simulink model "RBG_einMassenmodell_Versuchsplanung"  (Simulink 9.0)
settings: Solver=ode45  StartTime=0.0  StopTime=30  MaxStep=0.02  RelTol=1e-3  EnableMultiTasking=on
values from neighbouring files (symbols this model uses):
  hubMatlab = hubTest(k)    [generateErgebniseTabelle.m]    (also in simData.mat = 22)
  lastMatlab = masseTest(j)    [generateErgebniseTabelle.m]    (also in simData.mat = 560)
  zeitMatlab = zeitTest(l)    [generateErgebniseTabelle.m]    (also in simData.mat = 30)
libraries: simulink x1
settings Model: SuppressorTable=22 serialization::archive 11 0 6 0 0 0 11 0  Creator=beck  LastModifiedBy=jens
settings DataIOCC: LimitDataPoints=on  SignalLoggingSaveFormat=ModelDataLogs
settings OptimizationCC: ExpressionDepthLimit=2147483647  InitFltsAndDblsToZero=on
settings DebuggingCC: SaveWithParameterizedLinksMsg=none  SignalResolutionControl=TryResolveAllWithWarning  SolverPrmCheckMsg=warning  FcnCallInpInsideContextMsg=warning  StateNameClashWarn=warning  StrictBusMsg=Warning
settings GRTTargetCC: TargetFcnLib=ansi_tfl_tmw.mat  GeneratePreprocessorConditionals=Disable all  CombineOutputUpdateFcns=off  GRTInterface=on

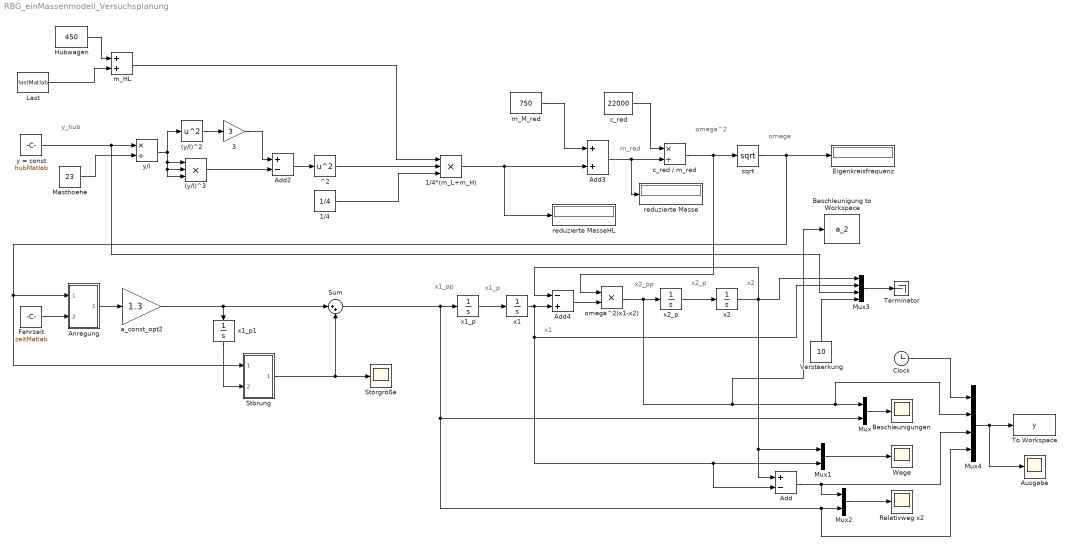
== system RBG_einMassenmodell_Versuchsplanung ==
  note: y_hub
  note: m_red
  note: omega^2
  note: x1_pp
  note: x2_pp
  note: x2_p
  note: x1_p
  note: omega
  note: x2
  note: x1
  (y/l)^2 : Math  Operator=square  SaturateOnIntegerOverflow=on
  (y/l)^3 : Product  Inputs=3  RndMeth=Zero
  1/4 : Constant  Value=1/4
  1/4*(m_L+m_H) : Product  Inputs=3  RndMeth=Zero
  3 : Gain  Gain=3
  Add : Sum  Inputs=+-
  Add2 : Sum  Inputs=+-
  Add3 : Sum
  Add4 : Sum  Inputs=-+
  Anregung : Subsystem
  Ausgabe : Scope
  Beschleunigung to Workspace : ToWorkspace  VariableName=a_2  SampleTime=-1
      settings: Save2DSignal=2-D array (concatenate along first dimension)
  Beschleunigungen : Scope
  Clock : Clock
  Eigenkreisfrequenz : Display
  Fahrzeit : Constant  Value=zeitMatlab
  Hubwagen : Constant  Value=450
  Last : Constant  Value=lastMatlab
  Masthoehe : Constant  Value=23
  Mux : Mux  Inputs=2
  Mux1 : Mux  Inputs=2
  Mux2 : Mux  Inputs=2
  Mux3 : Mux
  Mux4 : Mux
  Relativweg x2 : Scope
  Störgröße : Scope
  Störung : Subsystem
  Sum : Sum  Inputs=|++
  Terminator : Terminator
  To Workspace : ToWorkspace  VariableName=y  SampleTime=-1
  Verstaerkung : Constant  Value=10
  Wege : Scope
  ^2 : Math  Operator=square  SaturateOnIntegerOverflow=on
  a_const_opt2 : Gain  Gain=1.3
  c_red : Constant  Value=22000
  c_red / m_red : Product  Inputs=*/  RndMeth=Zero
  m_HL : Sum
  m_M_red : Constant  Value=750
  omega^2(x1-x2) : Product  RndMeth=Zero
  reduzierte Masse : Display
  reduzierte MasseHL : Display
  sqrt : Math  Operator=sqrt  SaturateOnIntegerOverflow=on
  x1 : Integrator
  x1_p : Integrator
  x1_p1 : Integrator
  x2 : Integrator
  x2_p : Integrator
  y = const : Constant  Value=hubMatlab
  y/l : Product  Inputs=*/  RndMeth=Zero
  wires:
  y = const/1 -> y/l/1, Mux3/3
  Mux/1 -> Beschleunigungen/1
  Mux1/1 -> Wege/1
  Masthoehe/1 -> y/l/2
  (y/l)^2/1 -> 3/1
  3/1 -> Add2/1
  (y/l)^3/1 -> Add2/2
  y/l/1 -> (y/l)^3/1, (y/l)^3/2, (y/l)^3/3, (y/l)^2/1
  c_red/1 -> c_red / m_red/1
  c_red / m_red/1 -> sqrt/1, omega^2(x1-x2)/1
  Add3/1 -> reduzierte Masse/1, c_red / m_red/2
  sqrt/1 -> Eigenkreisfrequenz/1, Störung/1(In1), Anregung/1(In1)
  omega^2(x1-x2)/1 -> x2_p/1, Beschleunigung to Workspace/1, Mux/1, Mux4/2
  x2_p/1 -> x2/1
  x1_p/1 -> x1/1
  Add4/1 -> omega^2(x1-x2)/2
  x1/1 -> Add4/2, Mux1/2, Add/2, Mux3/2
  x2/1 -> Mux1/1, Add/1, Mux3/1, Add4/1
  Verstaerkung/1 -> Mux3/4
  Add2/1 -> ^2/1
  m_M_red/1 -> Add3/1
  Mux2/1 -> Relativweg x2/1
  Add/1 -> Mux4/3, Mux2/1
  Last/1 -> m_HL/2
  Hubwagen/1 -> m_HL/1
  1/4*(m_L+m_H)/1 -> Add3/2, reduzierte MasseHL/1
  ^2/1 -> 1/4*(m_L+m_H)/2
  m_HL/1 -> 1/4*(m_L+m_H)/1
  1/4/1 -> 1/4*(m_L+m_H)/3
  Sum/1 -> x1_p/1, Mux/2, Mux2/2, Mux4/4
  Anregung/1(Out1) -> a_const_opt2/1
  Störung/1(Out1) -> Störgröße/1, Sum/2
  Clock/1 -> Mux4/1
  Mux4/1 -> To Workspace/1, Ausgabe/1
  a_const_opt2/1 -> Sum/1, x1_p1/1
  x1_p1/1 -> Störung/2(In2)
  Mux3/1 -> Terminator/1
  Fahrzeit/1 -> Anregung/2(In2)

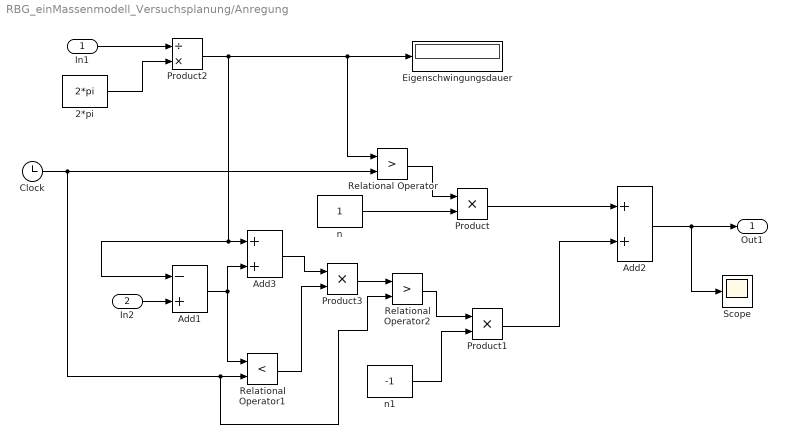
== system RBG_einMassenmodell_Versuchsplanung/Anregung ==
  In1 : Inport
  In2 : Inport  Port=2
  2*pi : Constant  Value=2*pi
  Add1 : Sum  Inputs=-+
  Add2 : Sum
  Add3 : Sum
  Clock : Clock
  Eigenschwingungsdauer : Display
  Product : Product  RndMeth=Zero
  Product1 : Product  RndMeth=Zero
  Product2 : Product  Inputs=/*  RndMeth=Zero
  Product3 : Product  RndMeth=Zero
  Relational Operator : RelationalOperator  Operator=>  RndMeth=Nearest
  Relational Operator1 : RelationalOperator  Operator=<  RndMeth=Nearest
  Relational Operator2 : RelationalOperator  Operator=>  RndMeth=Nearest
  Scope : Scope
  n : Constant
  n1 : Constant  Value=-1
  Out1 : Outport
  wires:
  2*pi/1 -> Product2/2
  Clock/1 -> Relational Operator/2, Relational Operator2/2, Relational Operator1/2
  n/1 -> Product/2
  Product2/1 -> Eigenschwingungsdauer/1, Relational Operator/1, Add1/1, Add3/1
  Relational Operator/1 -> Product/1
  In1/1 -> Product2/1
  Add2/1 -> Out1/1, Scope/1
  Product/1 -> Add2/1
  n1/1 -> Product1/2
  Relational Operator2/1 -> Product1/1
  Add3/1 -> Product3/1
  Relational Operator1/1 -> Product3/2
  Product3/1 -> Relational Operator2/1
  Product1/1 -> Add2/2
  In2/1 -> Add1/2
  Add1/1 -> Relational Operator1/1, Add3/2

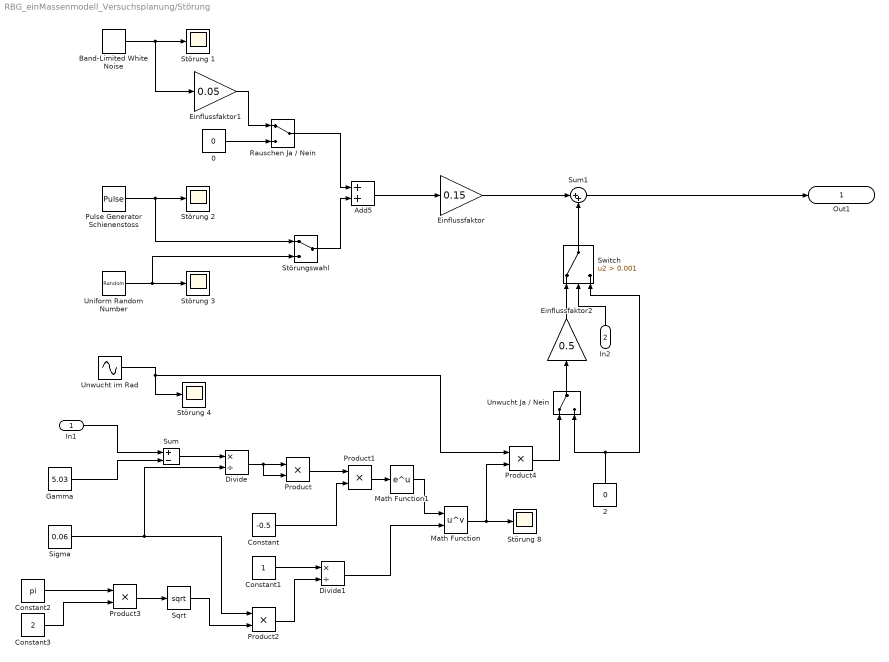
== system RBG_einMassenmodell_Versuchsplanung/Störung ==
  In1 : Inport
  In2 : Inport  Port=2
  0 : Constant  Value=0
  2 : Constant  Value=0
  Add5 : Sum
  Band-Limited White Noise : simulink/Sources/Band-Limited White Noise  Cov=[0.1]  Ts=0.1  seed=[23341]
  Constant : Constant  Value=-0.5
  Constant1 : Constant
  Constant2 : Constant  Value=pi
  Constant3 : Constant  Value=2
  Divide : Product  Inputs=*/
  Divide1 : Product  Inputs=*/
  Einflussfaktor : Gain  Gain=0.15
  Einflussfaktor1 : Gain  Gain=0.05
  Einflussfaktor2 : Gain  Gain=0.5
  Gamma : Constant  Value=5.03
  Math Function : Math  Operator=pow  SaturateOnIntegerOverflow=on
  Math Function1 : Math  SaturateOnIntegerOverflow=on
  Product{,1..4} (5 alike) : Product  RndMeth=Zero
  Pulse Generator Schienenstoss : DiscretePulseGenerator  PulseType=Time based  Amplitude=-1  Period=4
  Rauschen Ja / Nein : ManualSwitch
  Sigma : Constant  Value=0.06
  Sqrt : Sqrt  SaturateOnIntegerOverflow=on
  Störung {1..4,8} (5 alike) : Scope
  Störungswahl : ManualSwitch
  Sum : Sum  Inputs=+-
  Sum1 : Sum  Inputs=|++
  Switch : Switch  Criteria=u2 > Threshold  Threshold=0.001
  Uniform Random Number : UniformRandomNumber  SampleTime=1
  Unwucht Ja / Nein : ManualSwitch
  Unwucht im Rad : Sin  Frequency=5  SampleTime=0
  Out1 : Outport
  wires:
  Pulse Generator Schienenstoss/1 -> Störung 2/1, Störungswahl/1
  Add5/1 -> Einflussfaktor/1
  Band-Limited White Noise/1 -> Störung 1/1, Einflussfaktor1/1
  Störungswahl/1 -> Add5/2
  Uniform Random Number/1 -> Störung 3/1, Störungswahl/2
  Rauschen Ja / Nein/1 -> Add5/1
  Unwucht im Rad/1 -> Störung 4/1, Product4/1
  Gamma/1 -> Sum/2
  Sum/1 -> Divide/1
  Sigma/1 -> Divide/2, Product2/1
  Divide/1 -> Product/1, Product/2
  Product/1 -> Product1/1
  Constant/1 -> Product1/2
  Constant1/1 -> Divide1/1
  Constant2/1 -> Product3/1
  Constant3/1 -> Product3/2
  Product3/1 -> Sqrt/1
  Sqrt/1 -> Product2/2
  Product2/1 -> Divide1/2
  Math Function/1 -> Product4/2, Störung 8/1
  Product1/1 -> Math Function1/1
  Math Function1/1 -> Math Function/1
  Divide1/1 -> Math Function/2
  2/1 -> Switch/3, Unwucht Ja / Nein/2
  Product4/1 -> Unwucht Ja / Nein/1
  In1/1 -> Sum/1
  Einflussfaktor/1 -> Sum1/1
  Unwucht Ja / Nein/1 -> Einflussfaktor2/1
  Sum1/1 -> Out1/1
  Einflussfaktor2/1 -> Switch/1
  In2/1 -> Switch/2
  Switch/1 -> Sum1/2
  Einflussfaktor1/1 -> Rauschen Ja / Nein/1
  0/1 -> Rauschen Ja / Nein/2
